simulink model "WTPLoop"  (R2020a)
settings: Solver=ode4  StartTime=0.0  StopTime=200  FixedStep=0.1  RelTol=1e-3
values from neighbouring files (symbols this model uses):
  alpha = 0.018    [ParetoWTP.mat]    (also in WTPInit.m; WTPOP.m; sfun_WTP.m = param(5))
  beta = 0.2    [ParetoWTP.mat]    (also in WTPInit.m; WTPOP.m; sfun_WTP.m = param(3))
  D0 = 0.025    [ParetoWTP.mat]    (also in WTPInit.m)
  DO0 = 5    [ParetoWTP.mat]    (also in WTPInit.m)
  DOin0 = 0.5    [ParetoWTP.mat]    (also in WTPInit.m)
  DOmax = 10    [ParetoWTP.mat]    (also in WTPInit.m; WTPOP.m; sfun_WTP.m = param(9))
  K0 = 0.5    [ParetoWTP.mat]    (also in WTPInit.m; WTPOP.m; sfun_WTP.m = param(8))
  KDO = 2    [ParetoWTP.mat]    (also in WTPInit.m; WTPOP.m; sfun_WTP.m = param(4))
  Ks = 100    [ParetoWTP.mat]    (also in WTPInit.m; WTPOP.m; sfun_WTP.m = param(7))
  Qair0 = 27.5735    [ParetoWTP.mat]    (also in WTPInit.m)
  r = 0.6    [ParetoWTP.mat]    (also in WTPInit.m; WTPOP.m; sfun_WTP.m = param(2))
  S0 = 10.2941    [ParetoWTP.mat]    (also in WTPInit.m)
  Sin0 = 200    [ParetoWTP.mat]    (also in WTPInit.m)
  umax = 0.15    [ParetoWTP.mat]    (also in WTPInit.m; WTPOP.m; sfun_WTP.m = param(6))
  X0 = 298.2353    [ParetoWTP.mat]    (also in WTPInit.m)
  Xr0 = 596.4706    [ParetoWTP.mat]    (also in WTPInit.m)
  Y = 0.65    [ParetoWTP.mat]    (also in WTPInit.m; WTPOP.m; sfun_WTP.m = param(1))
libraries: simulink x1
settings Model: Creator=david  LastModifiedBy=david

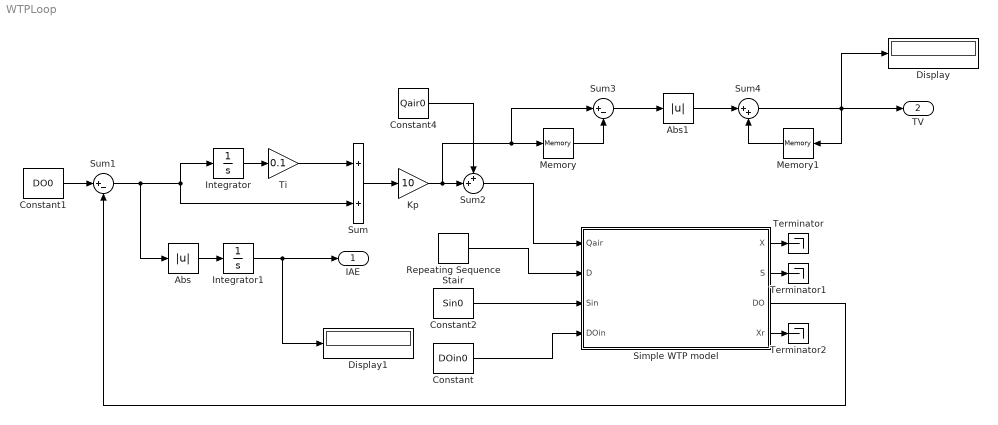
== system WTPLoop ==
  Abs : Abs
  Abs1 : Abs
  Constant : Constant  Value=DOin0
  Constant1 : Constant  Value=DO0
  Constant2 : Constant  Value=Sin0
  Constant4 : Constant  Value=Qair0
  Display : Display
  Display1 : Display
  Integrator : Integrator
  Integrator1 : Integrator
  Kp : Gain  Gain=10
  Memory : Memory
  Memory1 : Memory
  Repeating Sequence Stair : simulink/Sources/Repeating Sequence Stair  OutValues=[D0 0.5*D0 D0 1.5*D0].'  tsamp=20  OutMin=[]  OutMax=[]  OutDataTypeStr=double  OutputDataTypeScalingMode=double  OutDataType=fixdt(0,8)  ConRadixGroup=Best Precision: Vector-wise  OutScaling=2^-12
  Simple WTP model : Subsystem  mask{Y=Y, r=r, beta=beta, KDO=KDO, alpha=alpha, umax=umax, Ks=Ks, K0=K0, DOmax=DOmax, X0=X0, S0=S0, DO0=DO0, Xr0=Xr0}
      mask prompts: Y "Y ="; r "r ="; beta "beta ="; KDO "KDO ="; alpha "alpha ="; umax "umax ="; Ks "Ks ="; K0 "K0 ="; DOmax "DOmax ="; X0 "X ="; S0 "S ="; DO0 "DO ="; Xr0 "Xr ="
      mask DialogControl DescGroupVar Prompt: Simple WTP
      mask DialogControl DescTextVar Prompt: Fourth order non-linear WTP model
      mask DialogControl Container3 Prompt: Initial state
      mask Display: image('WTPFigure.png'); % Use "Edit Image" on toolstrip to change.
  Sum : Sum
  Sum1 : Sum  Inputs=|+-
  Sum2 : Sum  Inputs=++|
  Sum3 : Sum  Inputs=|+-
  Sum4 : Sum  Inputs=|++
  Terminator : Terminator
  Terminator1 : Terminator
  Terminator2 : Terminator
  Ti : Gain  Gain=0.1
  IAE : Outport
  TV : Outport  Port=2
  wires:
  Constant2/1 -> Simple WTP model/3(Sin)
  Constant/1 -> Simple WTP model/4(DOin)
  Simple WTP model/1(X) -> Terminator/1
  Simple WTP model/2(S) -> Terminator1/1
  Simple WTP model/4(Xr) -> Terminator2/1
  Integrator/1 -> Ti/1
  Constant1/1 -> Sum1/1
  Simple WTP model/3(DO) -> Sum1/2
  Sum1/1 -> Abs/1, Integrator/1, Sum/2
  Ti/1 -> Sum/1
  Sum/1 -> Kp/1
  Kp/1 -> Memory/1, Sum3/1, Sum2/2
  Constant4/1 -> Sum2/1
  Sum2/1 -> Simple WTP model/1(Qair)
  Abs/1 -> Integrator1/1
  Integrator1/1 -> Display1/1, IAE/1
  Repeating Sequence Stair/1 -> Simple WTP model/2(D)
  Memory/1 -> Sum3/2
  Sum3/1 -> Abs1/1
  Abs1/1 -> Sum4/1
  Sum4/1 -> Display/1, TV/1, Memory1/1
  Memory1/1 -> Sum4/2

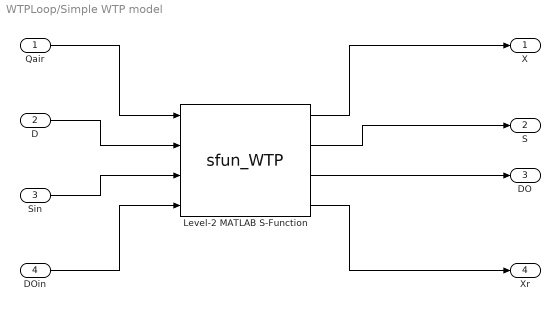
== system WTPLoop/Simple WTP model ==
  Qair : Inport
  D : Inport  Port=2
  Sin : Inport  Port=3
  DOin : Inport  Port=4
  Level-2 MATLAB S-Function : M-S-Function  FunctionName=sfun_WTP  Parameters=|
      | [Y;
      | r;
      | beta;
      | KDO;alpha;
      | umax; Ks; K0;
      | DOmax], [X0;S0;DO0;Xr0]
  X : Outport
  S : Outport  Port=2
  DO : Outport  Port=3
  Xr : Outport  Port=4
  wires:
  Sin/1 -> Level-2 MATLAB S-Function/3
  Level-2 MATLAB S-Function/2 -> S/1
  Level-2 MATLAB S-Function/1 -> X/1
  Qair/1 -> Level-2 MATLAB S-Function/1
  D/1 -> Level-2 MATLAB S-Function/2
  Level-2 MATLAB S-Function/4 -> Xr/1
  DOin/1 -> Level-2 MATLAB S-Function/4
  Level-2 MATLAB S-Function/3 -> DO/1
